simulink model "OmniWheelModel"  (R2018a)
settings: Solver=VariableStepAuto  StartTime=0.0  StopTime=10.0  RelTol=1e-3
libraries: simulink x2
settings Model: Creator=kartik  LastModifiedBy=kartik

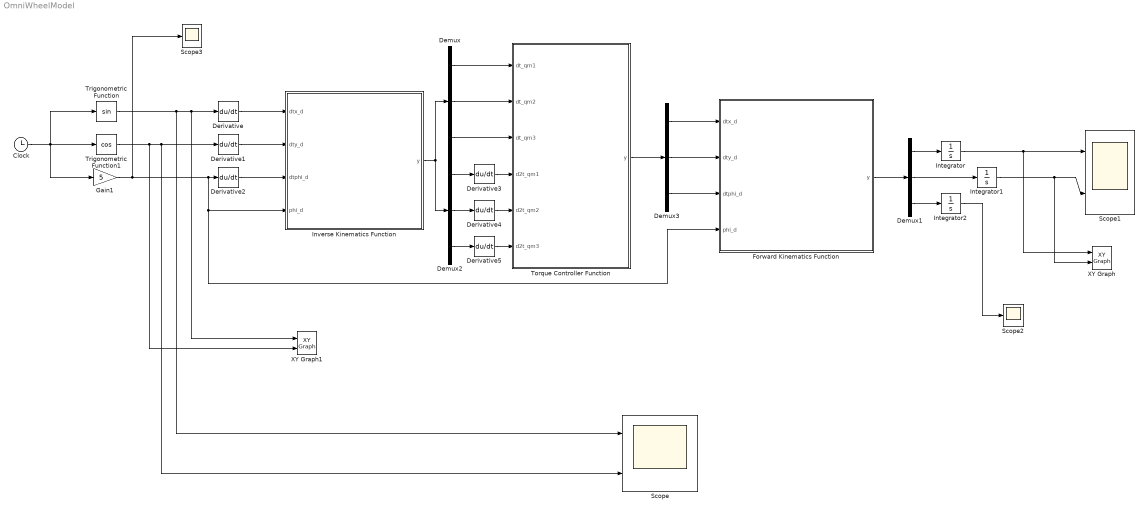
== system OmniWheelModel ==
  Clock : Clock
  Demux{,1..3} (4 alike) : Demux  Outputs=3
  Derivative{,1..5} (6 alike) : Derivative
  Forward Kinematics Function : MATLAB Function  TreatAsAtomicUnit=on
  Gain1 : Gain  Gain=5
  Integrator : Integrator
  Integrator1 : Integrator
  Integrator2 : Integrator
  Inverse Kinematics Function : MATLAB Function  TreatAsAtomicUnit=on
  Scope : Scope  NumInputPorts=2
  Scope1 : Scope  NumInputPorts=2
  Scope2 : Scope
  Scope3 : Scope
  Torque Controller Function : MATLAB Function  TreatAsAtomicUnit=on
  Trigonometric Function : Trigonometry
  Trigonometric Function1 : Trigonometry  Operator=cos
  XY Graph : simulink/Sinks/XY Graph  xmin=-0.00005  xmax=0.00005  ymin=-0.00005  ymax=0.00005  st=-1
  XY Graph1 : simulink/Sinks/XY Graph  xmin=-1  xmax=1  ymin=-1  ymax=1  st=-1
  wires:
  Inverse Kinematics Function/1(y) -> Demux2/1, Demux/1
  Forward Kinematics Function/1(y) -> Demux1/1
  Demux1/1 -> Integrator/1
  Demux1/2 -> Integrator1/1
  Demux1/3 -> Integrator2/1
  Clock/1 -> Trigonometric Function1/1, Gain1/1, Trigonometric Function/1
  Trigonometric Function/1 -> Scope/1, XY Graph1/1, Derivative/1
  Derivative/1 -> Inverse Kinematics Function/1(dtx_d)
  Derivative1/1 -> Inverse Kinematics Function/2(dty_d)
  Gain1/1 -> Scope3/1, Inverse Kinematics Function/4(phi_d), Forward Kinematics Function/4(phi_d), Derivative2/1
  Derivative2/1 -> Inverse Kinematics Function/3(dtphi_d)
  Demux/1 -> Torque Controller Function/1(dt_qm1)
  Demux/2 -> Torque Controller Function/2(dt_qm2)
  Demux/3 -> Torque Controller Function/3(dt_qm3)
  Demux2/1 -> Derivative3/1
  Demux2/2 -> Derivative4/1
  Demux2/3 -> Derivative5/1
  Derivative3/1 -> Torque Controller Function/4(d2t_qm1)
  Derivative4/1 -> Torque Controller Function/5(d2t_qm2)
  Derivative5/1 -> Torque Controller Function/6(d2t_qm3)
  Torque Controller Function/1(y) -> Demux3/1
  Demux3/1 -> Forward Kinematics Function/1(dtx_d)
  Demux3/2 -> Forward Kinematics Function/2(dty_d)
  Demux3/3 -> Forward Kinematics Function/3(dtphi_d)
  Integrator/1 -> XY Graph/1, Scope1/1
  Integrator1/1 -> XY Graph/2, Scope1/2
  Trigonometric Function1/1 -> XY Graph1/2, Scope/2, Derivative1/1
  Integrator2/1 -> Scope2/1

== matlab function OmniWheelModel/Forward Kinematics Function ==
  data: dtx_d input; y output; dty_d input; dtphi_d input; phi_d input
function y = OmniForwardKinematics(dtx_d, dty_d, dtphi_d, phi_d)
% Define Constants
r = 0.02; % Wheel Radius in m
L = 0.07; % Distance between center of robot to wheel in m
theta1 = 0; % In radians
theta2 = 2.0944;
theta3 = 4.18879;
% Geometrical Matrix
B = [-sin(theta1) -sin(theta2) -sin(theta3);
     cos(theta1) cos(theta2) cos(theta3);
     L L L]; 
% Rotational Matrix
R_wm = [cos(phi_d) sin(phi_d) 0;
        -sin(phi_d) cos(phi_d) 0;
        0 0 1];
% Reference Velocities
q_d = [dtx_d dty_d dtphi_d];
% Desired world coordinates
Xw = R_wm*(inv(B'))*(r*q_d');

y = Xw;

== matlab function OmniWheelModel/Inverse Kinematics Function ==
  data: dtx_d input; y output; dty_d input; dtphi_d input; phi_d input
function y = OmniInverseKinematics(dtx_d, dty_d, dtphi_d, phi_d)

% Define Constants
r = 0.02; % Wheel Radius in m
L = 0.07; % Distance between center of robot to wheel in m
theta1 = 0; % In radians
theta2 = 2.0944;
theta3 = 4.18879;
% Geometrical Matrix
B = [-sin(theta1) -sin(theta2) -sin(theta3);
     -cos(theta1) -cos(theta2) -cos(theta3);
     L L L]; 
% Rotational Matrix
R_wm = [cos(phi_d) sin(phi_d) 0;
        -sin(phi_d) cos(phi_d) 0;
        0 0 1];
% Desired world coordinates
Xw = [dtx_d dty_d dtphi_d];

% Generated velocities
q = (1/r)*(B')*(R_wm')*(Xw');

y = q;

== matlab function OmniWheelModel/Torque Controller Function ==
  data: dt_qm1 input; y output; dt_qm2 input; dt_qm3 input; d2t_qm1 input; d2t_qm2 input; d2t_qm3 input
function y = TorqueDynamics(dt_qm1, dt_qm2, dt_qm3, d2t_qm1, d2t_qm2, d2t_qm3)

% Define Constants
Jm = 2.7e-07;
Jl = 8e-5;
J = 4.6e-3;
r = 0.02;
L = 0.07;
n = 14;
m = 2.36;
Cm = 5e-8;
Cl = 0;

% Define Dynamic Parameters
k1 = Jm + (Jl/(n.^2)) + (((4*m*(L.^2) + J)*r.^2)/(9*L.^2*n.^2));
k2 = (((-2*m*(L.^2) + J)*r.^2)/(9*L.^2*n.^2));
k3 = Cm + (Cl/(n.^2));
k4 = (3.4641*m*r.^2)/(9*n.^2);
klr = 1/8.71;
km = 0.0144;
ke = 0.0145;

dt_phi = r*(dt_qm1 + dt_qm2 + dt_qm3)/(2*n*L);
dt_qm = [dt_qm1 dt_qm2 dt_qm3];
d2t_qm = [d2t_qm1 d2t_qm2 d2t_qm3];

% Coupled nonlinear equations of motion at actuator level
E = (k1/(klr*km))*[1 0 0; 0 1 0; 0 0 1]*d2t_qm' +... 
    (k2/(klr*km))*[0 1 1; 1 0 1; 1 1 0]*d2t_qm' + ...
    ((k3/klr*km) +ke)*[1 0 0; 0 1 0; 0 0 1]*dt_qm' + ...
    ((k4*dt_phi)/(klr*km))*[0 1 -1; -1 0 1; 1 -1 0]*dt_qm';

% Eqns pertaining to Torque Dynamics
Tm = (E - ke*(dt_qm'))*klr*km;
y = Tm;
